simulink model "ZsourceInverter"  (R2017b)
settings: Solver=ode45  StartTime=0.0  StopTime=0.1  MaxStep=1e-9  RelTol=1e-3  EnableMultiTasking=on
InitFcn:
  | Fs=100e3;
  | w=Fs*2*pi;
  | 
  | Vdc=100;
  | 
  | LP=200e-6;
  | LS=LP;
  | 
  | CP=1/w^2/LP;
  | CS=1/w^2/LS;
  | 
  | MPS=20e-6;
  | 
  | 
  | Rlp=0.1;
  | Rls=0.1;
libraries: powerlib x25, powerlib_meascontrol x10, simulink x4, peRmsMeasurement x1
settings Model: Creator=User  LastModifiedBy=SuperWindows
settings DataIOCC: LimitDataPoints=on  SaveFormat=Array
settings OptimizationCC: LifeSpan=inf
settings DebuggingCC: SolverPrmCheckMsg=warning  SFUnexpectedBacktrackingDiag=warning  SFNoUnconditionalDefaultTransitionDiag=warning  SFExecutionAtInitializationDiag=none
settings HardwareCC: ProdBitPerPointer=32  ProdBitPerSizeT=32  ProdBitPerPtrDiffT=32  ProdLargestAtomicFloat=None  ProdIntDivRoundTo=Undefined  ProdEndianess=Unspecified  ProdWordSize=32  ProdHWDeviceType=32-bit Generic
settings ModelReferenceCC: PropagateSignalLabelsOutOfModel=off
settings CodeAppCC: StateflowObjectComments=on
settings GRTTargetCC: TargetLangStandard=C89/C90 (ANSI)  GeneratePreprocessorConditionals=Disable all
settings ConfigComp: CovMetricSettings=dw  CovHtmlReporting=on  CovSaveCumulativeToWorkspaceVar=on  CovSaveSingleToWorkspaceVar=on  CovExternalEMLEnable=off  CovSFcnEnable=off
settings SimscapeCC: SimscapeNormalizeSystem=off

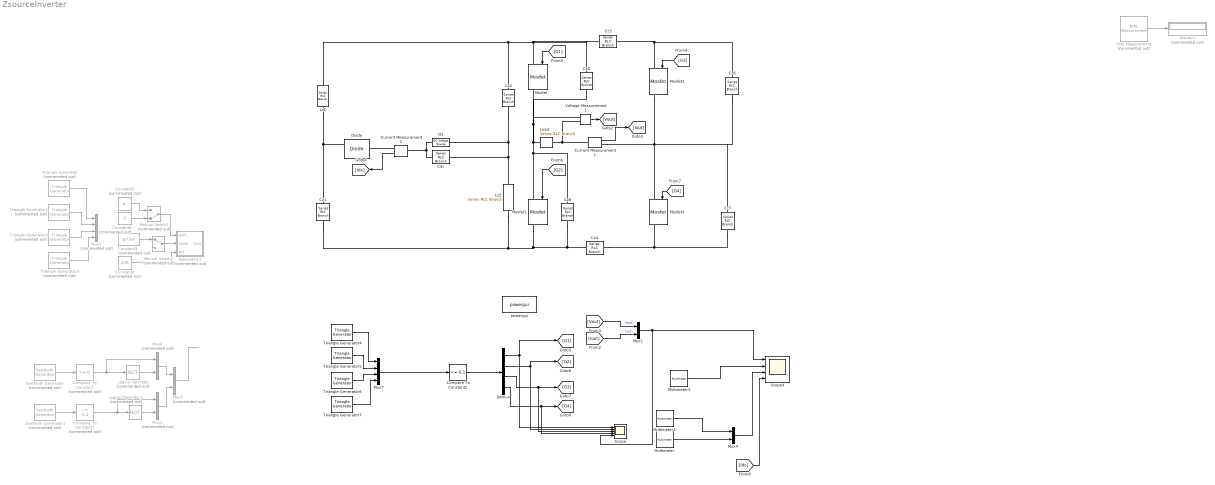
== system ZsourceInverter ==
  Cdc : powerlib/Elements/Series RLC Branch  LConnTagsString=__new0  RConnTagsString=__new0  BranchType=RC  Resistance=0.01  Inductance=1e-3  SetiL0=off  InitialCurrent=0  Capacitance=470e-6  Setx0=on  InitialVoltage=100  Measurements=Branch voltage and current
  Compare To Constant : simulink/Logic and Bit Operations/Compare To Constant  Commented=on  relop=>=  const=0  OutDataTypeStr=boolean
  Compare To Constant1 : simulink/Logic and Bit Operations/Compare To Constant  Commented=on  relop=>=  const=-0.2  OutDataTypeStr=boolean
  Compare To Constant2 : simulink/Logic and Bit Operations/Compare To Constant  relop=<=  const=0.1  OutDataTypeStr=boolean
  Constant3 : Constant  Commented=on  Value=pi*3/4
  Constant4 : Constant  Commented=on  Value=pi/6
  Constant5 : Constant  Commented=on  Value=pi
  Constant8 : Constant  Commented=on  Value=0
  Current Measurement1 : powerlib/Measurements/Current Measurement  PhasorSimulation=off  OutputType=Complex  PSBequivalent=0
  Current Measurement2 : powerlib/Measurements/Current Measurement  PhasorSimulation=off  OutputType=Complex  PSBequivalent=0
  Cz1 : powerlib/Elements/Series RLC Branch  LConnTagsString=__new0  RConnTagsString=__new0  BranchType=C  Resistance=1  Inductance=1e-3  SetiL0=off  InitialCurrent=0  Capacitance=470e-6  Setx0=on  InitialVoltage=130  Measurements=Branch voltage and current
  Cz2 : powerlib/Elements/Series RLC Branch  LConnTagsString=__new0  RConnTagsString=__new0  BranchType=C  Resistance=1  Inductance=1e-3  SetiL0=off  InitialCurrent=0  Capacitance=470e-6  Setx0=on  InitialVoltage=130  Measurements=Branch voltage and current
  Cz3 : powerlib/Elements/Series RLC Branch  LConnTagsString=__new0  RConnTagsString=__new0  BranchType=L  Resistance=1  Inductance=1e-7  SetiL0=off  InitialCurrent=0  Capacitance=470e-6  Setx0=on  InitialVoltage=130  Measurements=Branch voltage and current
  Cz4 : powerlib/Elements/Series RLC Branch  LConnTagsString=__new0  RConnTagsString=__new0  BranchType=L  Resistance=1  Inductance=1e-7  SetiL0=off  InitialCurrent=0  Capacitance=470e-6  Setx0=on  InitialVoltage=130  Measurements=Branch voltage and current
  Cz{5..8} (4 alike) : powerlib/Elements/Series RLC Branch  LConnTagsString=__new0  RConnTagsString=__new0  BranchType=RC  Resistance=10  Inductance=1e-7  SetiL0=off  InitialCurrent=0  Capacitance=33e-12  Setx0=on  InitialVoltage=130  Measurements=Branch voltage and current
  D1 : powerlib/Electrical Sources/DC Voltage Source  Amplitude=Vdc  Measurements=None
  Demux : Demux
  Diode : powerlib/Power Electronics/Diode  Ron=0.001  Lon=0  Vf=0.8  IC=0  UseSnubber=0  Rs=1e5  Cs=250e-9  Measurements=on
  Display1 : Display  Commented=on
  Load : powerlib/Elements/Series RLC Branch  LConnTagsString=__new0  RConnTagsString=__new0  BranchType=RLC  Resistance=10  Inductance=100e-6  SetiL0=off  InitialCurrent=0  Capacitance=25e-9  Setx0=on  InitialVoltage=60  Measurements=Branch voltage
  Logical Operator : Logic  Commented=on  Operator=NOT  AllPortsSameDT=off  OutDataTypeStr=boolean
  Logical Operator1 : Logic  Commented=on  Operator=NOT  AllPortsSameDT=off  OutDataTypeStr=boolean
  Lz1 : powerlib/Elements/Series RLC Branch  LConnTagsString=__new0  RConnTagsString=__new0  BranchType=L  Resistance=1  Inductance=1e-3  SetiL0=off  InitialCurrent=0  Capacitance=4700e-6  Setx0=on  InitialVoltage=60  Measurements=Branch voltage and current
  Lz2 : powerlib/Elements/Series RLC Branch  LConnTagsString=__new0  RConnTagsString=__new0  BranchType=L  Resistance=1  Inductance=1e-3  SetiL0=off  InitialCurrent=0  Capacitance=4700e-6  Setx0=on  InitialVoltage=60  Measurements=Branch voltage and current
  Manual Switch2 : ManualSwitch  Commented=on
  Manual Switch4 : ManualSwitch  Commented=on  CurrentSetting=0
  Mosfet{,1..3} (4 alike) : powerlib/Power Electronics/Mosfet  Ron=0.1  Lon=0  Rd=0.01  Vfd=0  IC=0  Rs=1e5  Cs=inf  Measurements=on
  Multimeter : powerlib/Measurements/Multimeter  PhasorSimulation=off  OutputType=Complex  sel=19  L=23  Gain=1  yselected={'Ib: Lz2'};  PSBOutputType=1  PSBequivalent=0  AxesSetting=[0,0.1,-100,100]  Display=0  SavedBlockNames=-11
  Multimeter1 : powerlib/Measurements/Multimeter  PhasorSimulation=off  OutputType=Complex  sel=18  L=23  Gain=1  yselected={'Ib: Lz1'};  PSBOutputType=1  PSBequivalent=0  AxesSetting=[0,0.1,-100,100]  Display=0  SavedBlockNames=-11
  Multimeter3 : powerlib/Measurements/Multimeter  PhasorSimulation=off  OutputType=Complex  sel=1  L=23  Gain=0  yselected={}  PSBOutputType=1  PSBequivalent=0  AxesSetting=[0,0.1,-100,100]  Display=0  SavedBlockNames=-11
  Mux1 : Mux  Inputs=2
  Mux2 : Mux  Commented=on
  Mux3 : Mux  Commented=on  Inputs=2
  Mux4 : Mux  Inputs=2
  Mux5 : Mux  Commented=on  Inputs=2
  Mux6 : Mux  Commented=on  Inputs=2
  Mux7 : Mux
  RMS Measurement : peRmsMeasurement/RMS Measurement  Commented=on  OverrideUsingVariant=Total  F=Fs  SpecifyHarmonics=off  K=[0 1 2]  Ts=1/Fs/100
  Sawtooth Generator : powerlib_meascontrol/Pulse & Signal Generators/Sawtooth Generator  Commented=on  Freq=100e3  Phase=0  Ts=0
      settings: SourceProductName=Simscape Power Systems
  Sawtooth Generator1 : powerlib_meascontrol/Pulse & Signal Generators/Sawtooth Generator  Commented=on  Freq=100e3  Phase=180  Ts=0
      settings: SourceProductName=Simscape Power Systems
  Scope : Scope  NumInputPorts=5
  Scope4 : Scope  NumInputPorts=4
  Subsystem2 : Subsystem  Commented=on  mask{f=100e3}
  Triangle Generator : powerlib_meascontrol/Pulse & Signal Generators/Triangle Generator  Commented=on  Freq=100e3  Phase=0  Ts=0
  Triangle Generator1 : powerlib_meascontrol/Pulse & Signal Generators/Triangle Generator  Commented=on  Freq=100e3  Phase=180  Ts=0
  Triangle Generator2 : powerlib_meascontrol/Pulse & Signal Generators/Triangle Generator  Commented=on  Freq=100e3  Phase=180-30  Ts=0
  Triangle Generator3 : powerlib_meascontrol/Pulse & Signal Generators/Triangle Generator  Commented=on  Freq=100e3  Phase=-30  Ts=0
  Triangle Generator4 : powerlib_meascontrol/Pulse & Signal Generators/Triangle Generator  Freq=100e3  Phase=0  Ts=0
  Triangle Generator5 : powerlib_meascontrol/Pulse & Signal Generators/Triangle Generator  Freq=100e3  Phase=180  Ts=0
  Triangle Generator6 : powerlib_meascontrol/Pulse & Signal Generators/Triangle Generator  Freq=100e3  Phase=180  Ts=0
  Triangle Generator7 : powerlib_meascontrol/Pulse & Signal Generators/Triangle Generator  Freq=100e3  Phase=0  Ts=0
  Voltage Measurement1 : powerlib/Measurements/Voltage Measurement  PhasorSimulation=off  OutputType=Complex  PSBequivalent=0
  powergui : powerlib/powergui  Priority=1  SimulationMode=Discrete  SampleTime=15e-9  frequency=60  Iterations=50  frequencyindice=0  Pbase=100e6  ErrMax=1e-4  UnitsV=kV  UnitsW=MW  buscounter=0  FunctionMessages=off  echomessages=off  EnableUseOfTLC=off  CurrentSourceSwitches=off  DisableSnubberDevices=off  DisableRonSwitches=off  DisableVfSwitches=off  DisplayEquations=off  SolverType=Tustin/Backward Euler (TBE)  Interpol=off  ExternalGateDelay=off  methode=off  Ts=100  x0status=blocks  SPID=on  SwTol=0  HookPort=off  RestoreLinks=warning  ResistiveCurrentMeasurement=off  Frange=[0:2:500]  Ylog=off  Xlog=on  ShowGrid=off  save=off  variable=ZData  structure=ScopeData2  ZoomFFT=off  StartTime=0.03  cycles=100  DisplayStyle=2  fundamental=100000  FreqAxis=off  MaxFrequency=100000*100  frequencyindicesteady=1  RmsSteady=1  display=off
  wires:
  Mux1/1 -> Scope/5, Scope4/1
  Mux4/1 -> Scope4/3
  RMS Measurement/1 -> Display1/1
  Voltage Measurement1/1 -> [Vout]
  Current Measurement1/1 -> [Iout]
  [Iout] -> Mux1/2  "Iout"
  [Vout] -> Mux1/1  "Vout"
  [G1] -> Mosfet/1
  [G4] -> Mosfet3/1
  [G2] -> Mosfet1/1
  [G3] -> Mosfet2/1
  Current Measurement2/1 -> [Idc]
  [Idc] -> Scope4/4
  Constant5/1 -> Manual Switch4/1
  Manual Switch4/1 -> Subsystem2/1(shift)
  Constant8/1 -> Manual Switch4/2
  Manual Switch2/1 -> Subsystem2/2("alpha ")
  Constant3/1 -> Manual Switch2/1
  Constant4/1 -> Subsystem2/3(Dst)
  Demux/1 -> [G1], Scope/1
  Demux/2 -> [G2], Scope/2
  Demux/3 -> Scope/3, [G3]
  Demux/4 -> Scope/4, [G4]
  Multimeter/1 -> Mux4/2
  Multimeter1/1 -> Mux4/1
  Triangle Generator/1 -> Mux2/1
  Triangle Generator1/1 -> Mux2/2
  Triangle Generator2/1 -> Mux2/3
  Triangle Generator3/1 -> Mux2/4
  Multimeter3/1 -> Scope4/2
  Triangle Generator7/1 -> Mux7/4
  Triangle Generator6/1 -> Mux7/3
  Triangle Generator5/1 -> Mux7/2
  Triangle Generator4/1 -> Mux7/1
  Sawtooth Generator1/1 -> Compare To Constant1/1
  Mux5/1 -> ?
  Compare To Constant/1 -> Mux6/1, Logical Operator/1
  Mux3/1 -> Mux5/2
  Logical Operator/1 -> Mux6/2
  Compare To Constant1/1 -> Mux3/1, Logical Operator1/1
  Sawtooth Generator/1 -> Compare To Constant/1
  Logical Operator1/1 -> Mux3/2
  Mux6/1 -> Mux5/1
  Mux7/1 -> Compare To Constant2/1
  Compare To Constant2/1 -> Demux/1
  connections:
  Mosfet1/LConn1 -- Cz8/LConn1 -- Load/RConn1 -- Voltage Measurement1/LConn1 -- Cz5/RConn1 -- Mosfet/RConn1
  Load/LConn1 -- Current Measurement1/LConn1 -- Voltage Measurement1/LConn2
  Cz2/RConn1 -- Lz2/LConn1 -- Cdc/RConn1 -- D1/LConn1
  Lz1/LConn1 -- Cz1/LConn1 -- Diode/RConn1
  Cz2/LConn1 -- Lz1/RConn1 -- Cz5/LConn1 -- Cz3/RConn1 -- Mosfet/LConn1
  Cz4/LConn1 -- Cz7/RConn1 -- Mosfet3/RConn1
  Mosfet2/RConn1 -- Cz7/LConn1 -- Cz6/RConn1 -- Current Measurement1/RConn1 -- Mosfet3/LConn1
  Cdc/LConn1 -- D1/RConn1 -- Current Measurement2/LConn1
  Diode/LConn1 -- Current Measurement2/RConn1
  Mosfet2/LConn1 -- Cz6/LConn1 -- Cz3/LConn1
  Cz1/RConn1 -- Lz2/RConn1 -- Mosfet1/RConn1 -- Cz4/RConn1 -- Cz8/RConn1

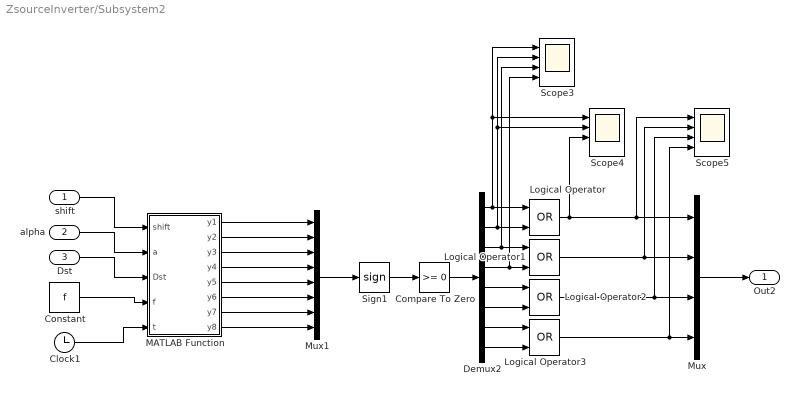
== system ZsourceInverter/Subsystem2 ==
  shift : Inport
  "alpha " : Inport  Port=2
  Dst : Inport  Port=3
  Clock1 : Clock
  Compare To Zero : simulink/Logic and Bit Operations/Compare To Zero  relop=>=  OutDataTypeStr=boolean
  Constant : Constant  Value=f
  Demux2 : Demux  Outputs=8
  Logical Operator{,1..3} (4 alike) : Logic  Operator=OR  AllPortsSameDT=off  OutDataTypeStr=boolean
  MATLAB Function : MATLAB Function  TreatAsAtomicUnit=on
  Mux : Mux
  Mux1 : Mux  Inputs=8
  Scope3 : Scope  NumInputPorts=4
  Scope4 : Scope  NumInputPorts=4
  Scope5 : Scope  NumInputPorts=4
  Sign1 : Signum
  Out2 : Outport
  wires:
  "alpha "/1 -> MATLAB Function/2(a)
  Clock1/1 -> MATLAB Function/5(t)
  MATLAB Function/1(y1) -> Mux1/1
  Mux/1 -> Out2/1
  MATLAB Function/2(y2) -> Mux1/2
  Mux1/1 -> Sign1/1
  shift/1 -> MATLAB Function/1(shift)
  Constant/1 -> MATLAB Function/4(f)
  MATLAB Function/3(y3) -> Mux1/3
  Dst/1 -> MATLAB Function/3(Dst)
  MATLAB Function/6(y6) -> Mux1/6
  MATLAB Function/7(y7) -> Mux1/7
  MATLAB Function/8(y8) -> Mux1/8
  MATLAB Function/5(y5) -> Mux1/5
  MATLAB Function/4(y4) -> Mux1/4
  Sign1/1 -> Compare To Zero/1
  Demux2/1 -> Logical Operator/1, Scope4/1, Scope3/1
  Demux2/2 -> Scope4/2, Scope3/2, Logical Operator/2
  Demux2/3 -> Scope3/3, Logical Operator1/1
  Demux2/4 -> Scope3/4, Logical Operator1/2
  Demux2/5 -> Logical Operator2/1
  Demux2/6 -> Logical Operator2/2
  Demux2/7 -> Logical Operator3/1
  Demux2/8 -> Logical Operator3/2
  Logical Operator/1 -> Scope4/3, Scope5/1, Mux/1
  Logical Operator1/1 -> Scope5/2, Mux/2
  Logical Operator2/1 -> Scope5/3, Mux/3
  Logical Operator3/1 -> Scope5/4, Mux/4
  Compare To Zero/1 -> Demux2/1

== matlab function ZsourceInverter/Subsystem2/MATLAB Function ==
  data: shift input; y1 output; a input; Dst input; f input; t input; y2 output; y3 output; y4 output; y5 output; y6 output; y7 output; y8 output
function [y1,y2,y3,y4,y5,y6,y7,y8] = fcn(shift,a,Dst,f,t)
w=2*pi*f;
if Dst>pi-a
    Dst=pi-a;
end
y1 = sin(w*t-a/2+shift);
y2 = sin(w*t-a/2+shift-Dst/2);

y3 = sin(w*t-a/2-pi+shift);
y4 = sin(w*t-a/2-pi+shift-Dst/2);

y5 = sin(w*t+a/2+shift);
y6 = sin(w*t+a/2+shift+Dst/2);

y7 = sin(w*t-pi+a/2+shift);
y8 = sin(w*t-pi+a/2+shift+Dst/2);




% y1 = sin(w*t+shift);
% y2 = sin(w*t+shift+Dst);
% y3 = sin(w*t+shift+pi);
% y4 = sin(w*t+shift+pi+Dst);
% y5 = sin(w*t+shift+pi+a);
% y6 = sin(w*t+shift+pi+a-Dst);
% y7 = sin(w*t+shift+a);
% y8 = sin(w*t+shift+a-Dst);
%#codegen
